simulink model "ExperimentThreeBD"  (R2015a)
settings: Solver=ode45  StartTime=0.0  StopTime=0.001  RelTol=1e-3
settings Model: Creator=Abdullah  LastModifiedBy=Abdullah

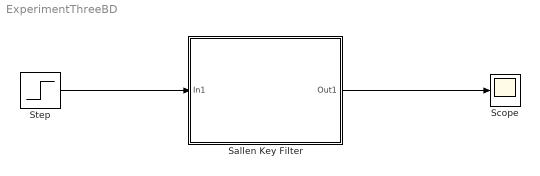
== system ExperimentThreeBD ==
  Sallen Key Filter : Subsystem
  Scope : Scope
  Step : Step  Time=0  SampleTime=0
  wires:
  Step/1 -> Sallen Key Filter/1(In1)
  Sallen Key Filter/1(Out1) -> Scope/1

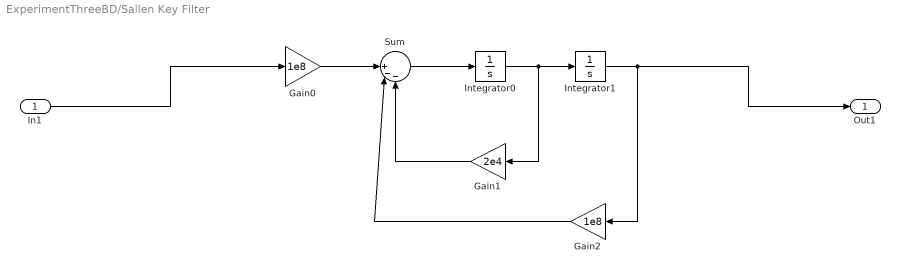
== system ExperimentThreeBD/Sallen Key Filter ==
  In1 : Inport
  Gain0 : Gain  Gain=1e8
  Gain1 : Gain  Gain=2e4
  Gain2 : Gain  Gain=1e8
  Integrator0 : Integrator
  Integrator1 : Integrator
  Sum : Sum  Inputs=||+--
  Out1 : Outport
  wires:
  In1/1 -> Gain0/1
  Gain2/1 -> Sum/2
  Integrator1/1 -> Out1/1, Gain2/1
  Gain1/1 -> Sum/3
  Gain0/1 -> Sum/1
  Sum/1 -> Integrator0/1
  Integrator0/1 -> Gain1/1, Integrator1/1
